simulink model "sedemo_ethernet"  (Simulink 7.5)
settings: Solver=VariableStepDiscrete  StartTime=0.0  StopTime=10.0  MaxStep=inf  RelTol=1e-3
PreLoadFcn:
  | MACInputSize = 25;
  | warning('off','MATLAB:divideByZero');
undefined symbols (not defined in the file or in its folder): des_subsystemblock, des_subsysteminport, des_subsystemoutport, des_subsystemsupportblock
libraries: simeventsrouting1 x30, simeventstranslate1 x26, simeventsattributes2 x16, simeventssink1 x13, simeventsserver1 x13, simeventsgenerators1 x11, simeventssignalmanage1 x9, simeventsgates1 x6, simeventsqueue1 x3, simeventsinfo x1
(part 2 of 5)

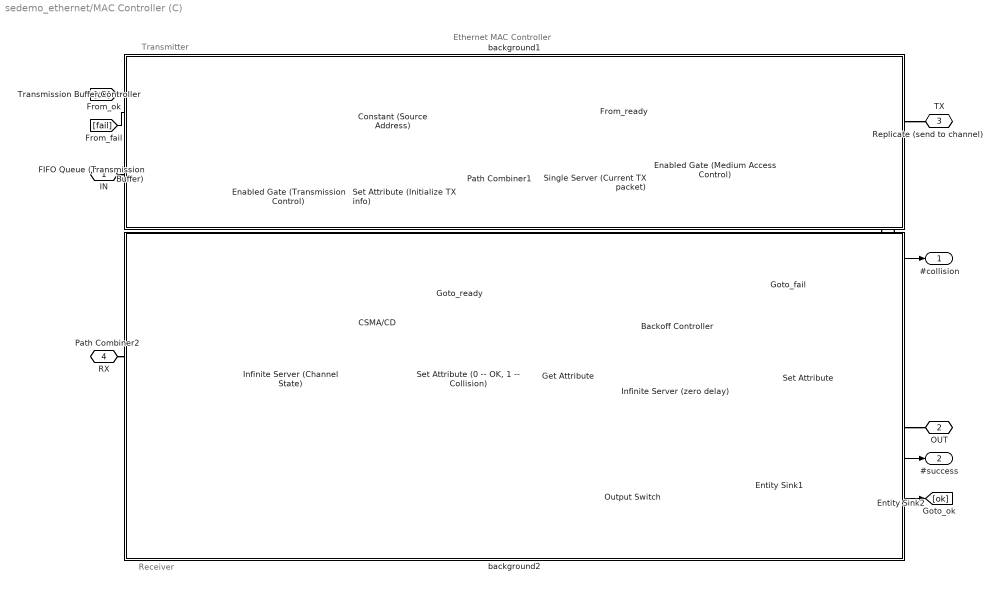
== system sedemo_ethernet/MAC Controller (C) ==
  note: Receiver
  note: Transmitter
  note: Ethernet MAC Controller
  Backoff Controller : Subsystem  LoadFcn=des_subsystemblock(gcb, 'load');  InitFcn=des_subsystemblock(gcb, 'init');  StartFcn=des_subsystemblock(gcb, 'start');  StopFcn=des_subsystemblock(gcb, 'stop');
      settings: CopyFcn=des_subsystemblock(gcb, 'copy');  DeleteFcn=des_subsystemblock(gcb, 'delete');  UndoDeleteFcn=des_subsystemblock(gcb, 'undodelete');  ModelCloseFcn=des_subsystemblock(gcb, 'modelclose');  PreSaveFcn=des_subsystemblock(gcb, 'presave');  NameChangeFcn=des_subsystemblock(gcb, 'namechange');  ParentCloseFcn=des_subsystemblock(gcb, 'parentclose');  ErrorFcn=des_error_redirect
  CSMA/CD : Subsystem
  Constant (Source Address) : Constant  Value=SrcAddress  OutDataType=sfix(16)  OutScaling=2^0
  Enabled Gate (Medium Access Control) : simeventsgates1/Enabled Gate  Priority=1  SystemSampleTime=-1  SpecifyEventPriority=off  PriorityGateEnableOpenClose=200  StatNumberDeparted=Off
  Enabled Gate (Transmission Control) : simeventsgates1/Enabled Gate  Priority=1  SystemSampleTime=-1  SpecifyEventPriority=off  PriorityGateEnableOpenClose=200  StatNumberDeparted=On
  Entity Sink1 : simeventssink1/Entity Sink  Priority=1  SystemSampleTime=-1  AvailableForArrivals=on  StatNumberArrived=On
  Entity Sink2 : simeventssink1/Entity Sink  Priority=1  SystemSampleTime=-1  AvailableForArrivals=on  StatNumberArrived=Off
  FIFO Queue (Transmission Buffer) : simeventsqueue1/FIFO Queue  Priority=1  SystemSampleTime=-1  Capacity=MACInputSize  EnableTOPort=off  StatNumberDeparted=Off  StatNumberInBlock=Off  StatPendingEntity=Off  StatAverageWait=Off  StatAverageQueueLength=Off  StatNumberTimedout=Off
  Get Attribute : simeventsattributes2/Get Attribute  Priority=1  DialogController=des_ddg_create  DialogControllerArgs=DataTag199  SystemSampleTime=-1  AttributeName=SrcAddress|NumCollision|Collision  AttributeMissing=Error|Error|Error  AttributeDefaultValue=0|0|0  AttributeSendTiming=After entity departure|After entity departure|After entity departure  AttributeTreatAsVector=1|1|1  StatNumberDeparted=Off  EvaluatedDefaultAttributeValue={[];[];[]}
  Infinite Server (Channel State) : simeventsserver1/Infinite Server  Priority=1  SystemSampleTime=-1  ServiceTimeFrom=Attribute  ServiceTime=1  AttributeName=ServiceTime  PriorityServiceCompletion=500  EnableTOPort=off  StatNumberDeparted=Off  StatNumberInBlock=On  StatPendingEntity=Off  StatNumberPending=Off  StatAverageWait=Off  StatNumberTimedout=Off
  Infinite Server (zero delay) : simeventsserver1/Infinite Server  Priority=1  SystemSampleTime=-1  ServiceTimeFrom=Dialog  ServiceTime=0  AttributeName=ServiceTime  PriorityServiceCompletion=200  EnableTOPort=off  StatNumberDeparted=Off  StatNumberInBlock=Off  StatPendingEntity=Off  StatNumberPending=Off  StatAverageWait=Off  StatNumberTimedout=Off
  Output Switch : simeventsrouting1/Output Switch  Priority=1  SystemSampleTime=-1  NumberOutputPorts=4  SwitchingCriterion=From attribute  InitialSeed=34567  AttributeName=Route  InitialConditionsOpt=off  InitialConditions=1  EntityBufferOpt=off  SpecifyEventPriority=off  PriorityOutputSwitchSelectPort=4100  TimeoutPortOpt=off  StatNumberDeparted=Off  StatNumberTimedOut=Off  StatPendingEntity=Off  StatLastDeparturePort=Off  EvaluatedNumPorts=4
  Path Combiner1 : simeventsrouting1/Path Combiner  Priority=1  SystemSampleTime=-1  NumberInputPorts=2  InputPortPrecedence=IN1 port  InitialSeed=45675  SpecifyEventPriority=off  PriorityPathCombinerPortPrecedenceSelection=4100  StatNumberDeparted=Off  StatLastArrivalPort=Off  EvaluatedNumPorts=2
  Path Combiner2 : simeventsrouting1/Path Combiner  Priority=1  SystemSampleTime=-1  NumberInputPorts=2  InputPortPrecedence=IN1 port  InitialSeed=45675  SpecifyEventPriority=off  PriorityPathCombinerPortPrecedenceSelection=4100  StatNumberDeparted=Off  StatLastArrivalPort=Off  EvaluatedNumPorts=2
  Replicate (send to channel) : simeventsrouting1/Replicate  Priority=1  SystemSampleTime=-1  NumberOutputPorts=2  ReplicateEntityWhen=All entity output ports are not blocked  OutputPortPrecedence=OUT1 port  InitialSeed=56789  ActionUponBlocking=Discard entity  StatNumberArrived=Off  StatNumberDeparted=Off  EvaluatedNumPorts=2
  Set Attribute : simeventsattributes2/Set Attribute  Priority=1  DialogController=des_ddg_create  DialogControllerArgs=DataTag207  SystemSampleTime=-1  AttributeFrom=Signal port|Signal port|Signal port  AttributeName=Route|NumCollision|BckoffTime  AttributeTreatAsVector=1|1|1  AttributeValue=0|0|0  AttributeCreate=on  StatNumberDeparted=Off  EvaluatedAttributeValue={[];[];[]}
  "Set Attribute (0 -- OK, 1 -- Collision)" : simeventsattributes2/Set Attribute  Priority=1  DialogController=des_ddg_create  DialogControllerArgs=DataTag209  SystemSampleTime=-1  AttributeFrom=Signal port  AttributeName=Collision  AttributeTreatAsVector=1  AttributeValue=0  AttributeCreate=on  StatNumberDeparted=Off  EvaluatedAttributeValue={[]}
  Set Attribute (Initialize TX info) : simeventsattributes2/Set Attribute  Priority=1  DialogController=des_ddg_create  DialogControllerArgs=DataTag211  SystemSampleTime=-1  AttributeFrom=Signal port|Dialog|Dialog  AttributeName=SrcAddress|BckoffTime|NumCollision  AttributeTreatAsVector=1|1|1  AttributeValue=0|0|0  AttributeCreate=on  StatNumberDeparted=Off  EvaluatedAttributeValue={[];0;0}
  Single Server (Current TX packet) : simeventsserver1/Single Server  Priority=1  SystemSampleTime=-1  ServiceTimeFrom=Attribute  ServiceTime=0  AttributeName=BckoffTime  PriorityServiceCompletion=500  PermitPreemption=off  SortingAttributeName=PriorityAttributeName  SortingDirection=Ascending  WriteToAttribute=off  ResidualAttributeName=ResidualServiceTime  CreateAttribute=on  EnableTOPort=off  StatNumberDeparted=Off  StatNumberInBlock=Off  StatNumberPreempted=Off  StatPendingEntity=Off  StatAverageWait=Off  StatUtilization=Off  StatNumberTimedout=Off
  Transmission Buffer Controller : Subsystem
  background1 : Subsystem
      mask Display: disp('')
  background2 : Subsystem
      mask Display: disp('')
  IN : PMIOPort  Port=1  Side=Right
  OUT : PMIOPort  Port=2  Side=Right
  TX : PMIOPort  Port=3  Side=Left
  RX : PMIOPort  Port=4  Side=Left
  #collision : Outport  OutDataType=sfix(16)  OutScaling=2^0
  #success : Outport  Port=2  OutDataType=sfix(16)  OutScaling=2^0
  wires:
  CSMA/CD/1(l_ready) -> [rdy]
  Backoff Controller/2(#failure) -> [fail]
  [fail] -> Transmission Buffer Controller/3(#failure)
  [ok] -> Transmission Buffer Controller/2(#success)
  [rdy] -> Enabled Gate (Medium Access Control)/1
  Backoff Controller/3(route) -> Set Attribute/1
  Backoff Controller/4(#collision1) -> Set Attribute/2
  Backoff Controller/5(bckoffTime) -> Set Attribute/3
  Backoff Controller/1(#sum) -> #collision/1
  Get Attribute/2 -> Backoff Controller/2(#collision)
  Get Attribute/3 -> Backoff Controller/3(collision)
  Get Attribute/1 -> Backoff Controller/1(SrcAddr)
  Constant (Source Address)/1 -> Set Attribute (Initialize TX info)/1
  Transmission Buffer Controller/1(state) -> Enabled Gate (Transmission Control)/1
  CSMA/CD/2(pck_ok) -> "Set Attribute (0 -- OK, 1 -- Collision)"/1
  Entity Sink1/1 -> [ok], #success/1
  Infinite Server (Channel State)/1 -> CSMA/CD/1(l_status)
  Enabled Gate (Transmission Control)/1 -> Transmission Buffer Controller/1(#tx)
  connections:
  Output Switch/RConn4 -- Path Combiner1/LConn1
  Output Switch/RConn1 -- OUT/RConn1
  Set Attribute/RConn1 -- Output Switch/LConn1
  "Set Attribute (0 -- OK, 1 -- Collision)"/RConn1 -- Get Attribute/LConn1
  Infinite Server (zero delay)/RConn1 -- Set Attribute/LConn1
  Get Attribute/RConn1 -- Infinite Server (zero delay)/LConn1
  Output Switch/RConn2 -- Entity Sink1/LConn1
  Output Switch/RConn3 -- Entity Sink2/LConn1
  Enabled Gate (Transmission Control)/RConn1 -- Set Attribute (Initialize TX info)/LConn1
  Set Attribute (Initialize TX info)/RConn1 -- Path Combiner1/LConn2
  Replicate (send to channel)/RConn1 -- TX/RConn1
  FIFO Queue (Transmission Buffer)/RConn1 -- Enabled Gate (Transmission Control)/LConn1
  Replicate (send to channel)/RConn2 -- Path Combiner2/LConn1
  Path Combiner1/RConn1 -- Single Server (Current TX packet)/LConn1
  RX/RConn1 -- Path Combiner2/LConn2
  Enabled Gate (Medium Access Control)/RConn1 -- Replicate (send to channel)/LConn1
  IN/RConn1 -- FIFO Queue (Transmission Buffer)/LConn1
  Infinite Server (Channel State)/RConn1 -- "Set Attribute (0 -- OK, 1 -- Collision)"/LConn1
  Path Combiner2/RConn1 -- Infinite Server (Channel State)/LConn1
  Single Server (Current TX packet)/RConn1 -- Enabled Gate (Medium Access Control)/LConn1

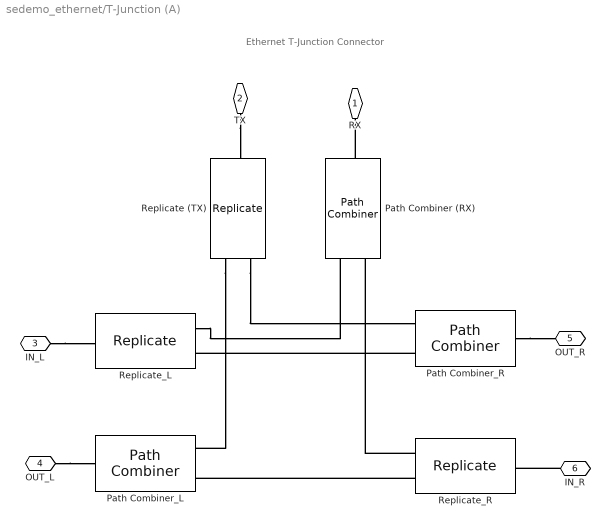
== system sedemo_ethernet/T-Junction (A) ==
  note: Ethernet T-Junction Connector
  Path Combiner (RX) : simeventsrouting1/Path Combiner  Priority=1  SystemSampleTime=-1  NumberInputPorts=2  InputPortPrecedence=IN1 port  InitialSeed=45675  SpecifyEventPriority=off  PriorityPathCombinerPortPrecedenceSelection=4100  StatNumberDeparted=Off  StatLastArrivalPort=Off  EvaluatedNumPorts=2
  Path Combiner_L : simeventsrouting1/Path Combiner  Priority=1  SystemSampleTime=-1  NumberInputPorts=2  InputPortPrecedence=IN1 port  InitialSeed=45675  SpecifyEventPriority=off  PriorityPathCombinerPortPrecedenceSelection=4100  StatNumberDeparted=Off  StatLastArrivalPort=Off  EvaluatedNumPorts=2
  Path Combiner_R : simeventsrouting1/Path Combiner  Priority=1  SystemSampleTime=-1  NumberInputPorts=2  InputPortPrecedence=IN1 port  InitialSeed=45675  SpecifyEventPriority=off  PriorityPathCombinerPortPrecedenceSelection=4100  StatNumberDeparted=Off  StatLastArrivalPort=Off  EvaluatedNumPorts=2
  Replicate (TX) : simeventsrouting1/Replicate  Priority=1  SystemSampleTime=-1  NumberOutputPorts=2  ReplicateEntityWhen=All entity output ports are not blocked  OutputPortPrecedence=OUT1 port  InitialSeed=56789  ActionUponBlocking=Discard entity  StatNumberArrived=Off  StatNumberDeparted=Off  EvaluatedNumPorts=2
  Replicate_L : simeventsrouting1/Replicate  Priority=1  SystemSampleTime=-1  NumberOutputPorts=2  ReplicateEntityWhen=All entity output ports are not blocked  OutputPortPrecedence=OUT1 port  InitialSeed=56789  ActionUponBlocking=Discard entity  StatNumberArrived=Off  StatNumberDeparted=Off  EvaluatedNumPorts=2
  Replicate_R : simeventsrouting1/Replicate  Priority=1  SystemSampleTime=-1  NumberOutputPorts=2  ReplicateEntityWhen=All entity output ports are not blocked  OutputPortPrecedence=OUT1 port  InitialSeed=56789  ActionUponBlocking=Discard entity  StatNumberArrived=Off  StatNumberDeparted=Off  EvaluatedNumPorts=2
  RX : PMIOPort  Port=1  Side=Right
  TX : PMIOPort  Port=2  Side=Left
  IN_L : PMIOPort  Port=3  Side=Left
  OUT_L : PMIOPort  Port=4  Side=Left
  OUT_R : PMIOPort  Port=5  Side=Right
  IN_R : PMIOPort  Port=6  Side=Right
  connections:
  Replicate (TX)/RConn1 -- Path Combiner_L/LConn1
  Replicate (TX)/RConn2 -- Path Combiner_R/LConn1
  TX/RConn1 -- Replicate (TX)/LConn1
  Path Combiner (RX)/RConn1 -- RX/RConn1
  Replicate_R/RConn2 -- Path Combiner_L/LConn2
  OUT_L/RConn1 -- Path Combiner_L/RConn1
  Replicate_R/RConn1 -- Path Combiner (RX)/LConn2
  Replicate_L/RConn1 -- Path Combiner (RX)/LConn1
  IN_R/RConn1 -- Replicate_R/LConn1
  Path Combiner_R/LConn2 -- Replicate_L/RConn2
  IN_L/RConn1 -- Replicate_L/LConn1
  Path Combiner_R/RConn1 -- OUT_R/RConn1

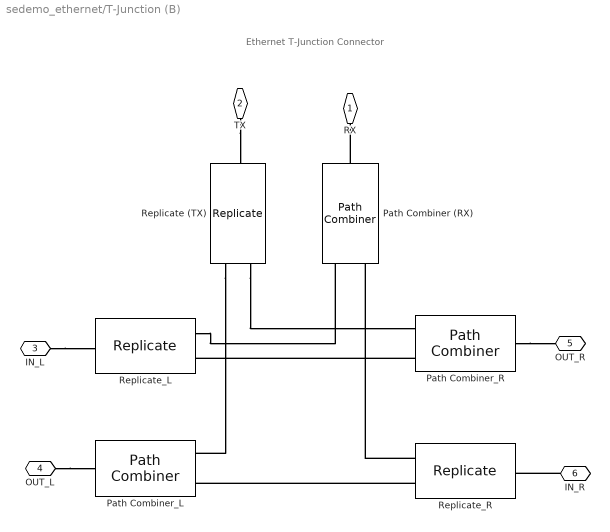
== system sedemo_ethernet/T-Junction (B) ==
  note: Ethernet T-Junction Connector
  Path Combiner (RX) : simeventsrouting1/Path Combiner  Priority=1  SystemSampleTime=-1  NumberInputPorts=2  InputPortPrecedence=IN1 port  InitialSeed=45675  SpecifyEventPriority=off  PriorityPathCombinerPortPrecedenceSelection=4100  StatNumberDeparted=Off  StatLastArrivalPort=Off  EvaluatedNumPorts=2
  Path Combiner_L : simeventsrouting1/Path Combiner  Priority=1  SystemSampleTime=-1  NumberInputPorts=2  InputPortPrecedence=IN1 port  InitialSeed=45675  SpecifyEventPriority=off  PriorityPathCombinerPortPrecedenceSelection=4100  StatNumberDeparted=Off  StatLastArrivalPort=Off  EvaluatedNumPorts=2
  Path Combiner_R : simeventsrouting1/Path Combiner  Priority=1  SystemSampleTime=-1  NumberInputPorts=2  InputPortPrecedence=IN1 port  InitialSeed=45675  SpecifyEventPriority=off  PriorityPathCombinerPortPrecedenceSelection=4100  StatNumberDeparted=Off  StatLastArrivalPort=Off  EvaluatedNumPorts=2
  Replicate (TX) : simeventsrouting1/Replicate  Priority=1  SystemSampleTime=-1  NumberOutputPorts=2  ReplicateEntityWhen=All entity output ports are not blocked  OutputPortPrecedence=OUT1 port  InitialSeed=56789  ActionUponBlocking=Discard entity  StatNumberArrived=Off  StatNumberDeparted=Off  EvaluatedNumPorts=2
  Replicate_L : simeventsrouting1/Replicate  Priority=1  SystemSampleTime=-1  NumberOutputPorts=2  ReplicateEntityWhen=All entity output ports are not blocked  OutputPortPrecedence=OUT1 port  InitialSeed=56789  ActionUponBlocking=Discard entity  StatNumberArrived=Off  StatNumberDeparted=Off  EvaluatedNumPorts=2
  Replicate_R : simeventsrouting1/Replicate  Priority=1  SystemSampleTime=-1  NumberOutputPorts=2  ReplicateEntityWhen=All entity output ports are not blocked  OutputPortPrecedence=OUT1 port  InitialSeed=56789  ActionUponBlocking=Discard entity  StatNumberArrived=Off  StatNumberDeparted=Off  EvaluatedNumPorts=2
  RX : PMIOPort  Port=1  Side=Right
  TX : PMIOPort  Port=2  Side=Left
  IN_L : PMIOPort  Port=3  Side=Left
  OUT_L : PMIOPort  Port=4  Side=Left
  OUT_R : PMIOPort  Port=5  Side=Right
  IN_R : PMIOPort  Port=6  Side=Right
  connections:
  Path Combiner_R/RConn1 -- OUT_R/RConn1
  IN_L/RConn1 -- Replicate_L/LConn1
  Path Combiner_R/LConn2 -- Replicate_L/RConn2
  IN_R/RConn1 -- Replicate_R/LConn1
  Replicate_L/RConn1 -- Path Combiner (RX)/LConn1
  Replicate_R/RConn1 -- Path Combiner (RX)/LConn2
  OUT_L/RConn1 -- Path Combiner_L/RConn1
  Replicate_R/RConn2 -- Path Combiner_L/LConn2
  Path Combiner (RX)/RConn1 -- RX/RConn1
  TX/RConn1 -- Replicate (TX)/LConn1
  Replicate (TX)/RConn2 -- Path Combiner_R/LConn1
  Replicate (TX)/RConn1 -- Path Combiner_L/LConn1

== system sedemo_ethernet/T-Junction (C) ==
  note: Ethernet T-Junction Connector
  Path Combiner (RX) : simeventsrouting1/Path Combiner  Priority=1  SystemSampleTime=-1  NumberInputPorts=2  InputPortPrecedence=IN1 port  InitialSeed=45675  SpecifyEventPriority=off  PriorityPathCombinerPortPrecedenceSelection=4100  StatNumberDeparted=Off  StatLastArrivalPort=Off  EvaluatedNumPorts=2
  Path Combiner_L : simeventsrouting1/Path Combiner  Priority=1  SystemSampleTime=-1  NumberInputPorts=2  InputPortPrecedence=IN1 port  InitialSeed=45675  SpecifyEventPriority=off  PriorityPathCombinerPortPrecedenceSelection=4100  StatNumberDeparted=Off  StatLastArrivalPort=Off  EvaluatedNumPorts=2
  Path Combiner_R : simeventsrouting1/Path Combiner  Priority=1  SystemSampleTime=-1  NumberInputPorts=2  InputPortPrecedence=IN1 port  InitialSeed=45675  SpecifyEventPriority=off  PriorityPathCombinerPortPrecedenceSelection=4100  StatNumberDeparted=Off  StatLastArrivalPort=Off  EvaluatedNumPorts=2
  Replicate (TX) : simeventsrouting1/Replicate  Priority=1  SystemSampleTime=-1  NumberOutputPorts=2  ReplicateEntityWhen=All entity output ports are not blocked  OutputPortPrecedence=OUT1 port  InitialSeed=56789  ActionUponBlocking=Discard entity  StatNumberArrived=Off  StatNumberDeparted=Off  EvaluatedNumPorts=2
  Replicate_L : simeventsrouting1/Replicate  Priority=1  SystemSampleTime=-1  NumberOutputPorts=2  ReplicateEntityWhen=All entity output ports are not blocked  OutputPortPrecedence=OUT1 port  InitialSeed=56789  ActionUponBlocking=Discard entity  StatNumberArrived=Off  StatNumberDeparted=Off  EvaluatedNumPorts=2
  Replicate_R : simeventsrouting1/Replicate  Priority=1  SystemSampleTime=-1  NumberOutputPorts=2  ReplicateEntityWhen=All entity output ports are not blocked  OutputPortPrecedence=OUT1 port  InitialSeed=56789  ActionUponBlocking=Discard entity  StatNumberArrived=Off  StatNumberDeparted=Off  EvaluatedNumPorts=2
  RX : PMIOPort  Port=1  Side=Right
  TX : PMIOPort  Port=2  Side=Left
  IN_L : PMIOPort  Port=3  Side=Left
  OUT_L : PMIOPort  Port=4  Side=Left
  OUT_R : PMIOPort  Port=5  Side=Right
  IN_R : PMIOPort  Port=6  Side=Right
  connections:
  Path Combiner_R/RConn1 -- OUT_R/RConn1
  IN_L/RConn1 -- Replicate_L/LConn1
  Path Combiner_R/LConn2 -- Replicate_L/RConn2
  IN_R/RConn1 -- Replicate_R/LConn1
  Replicate_L/RConn1 -- Path Combiner (RX)/LConn1
  Replicate_R/RConn1 -- Path Combiner (RX)/LConn2
  OUT_L/RConn1 -- Path Combiner_L/RConn1
  Replicate_R/RConn2 -- Path Combiner_L/LConn2
  Path Combiner (RX)/RConn1 -- RX/RConn1
  TX/RConn1 -- Replicate (TX)/LConn1
  Replicate (TX)/RConn2 -- Path Combiner_R/LConn1
  Replicate (TX)/RConn1 -- Path Combiner_L/LConn1

== system sedemo_ethernet/Terminator (L) ==
  note: Ethernet Terminator
  Entity Sink : simeventssink1/Entity Sink  Priority=1  SystemSampleTime=-1  AvailableForArrivals=on  StatNumberArrived=Off
  Event-Based Entity Generator : simeventsgenerators1/Entity Generators/Event-Based Entity Generator  Priority=1  DialogController=des_ddg_create  DialogControllerArgs=DataTag244  SystemSampleTime=-1  GenerateEntitiesUpon=Change in signal from port vc  SignalEdgeType=Rising  SpecifyEventPriority=off  PriorityEntityGeneration=300  GenerateEntityAtSimulationStart=on  AllowBlocking=on  ResponseDuringBlockage=Discard generated entities  EntityType=Standard  StatNumberDeparted=Off  StatPendingEntity=Off  StatAverageIntergenerationTime=Off
  Ground : Ground
  OUT : PMIOPort  Port=1  Side=Left
  IN : PMIOPort  Port=2  Side=Left
  wires:
  Ground/1 -> Event-Based Entity Generator/1
  connections:
  Event-Based Entity Generator/RConn1 -- OUT/RConn1
  IN/RConn1 -- Entity Sink/LConn1

== system sedemo_ethernet/Terminator (R) ==
  Entity Sink : simeventssink1/Entity Sink  Priority=1  SystemSampleTime=-1  AvailableForArrivals=on  StatNumberArrived=Off
  Event-Based Entity Generator : simeventsgenerators1/Entity Generators/Event-Based Entity Generator  Priority=1  DialogController=des_ddg_create  DialogControllerArgs=DataTag247  SystemSampleTime=-1  GenerateEntitiesUpon=Change in signal from port vc  SignalEdgeType=Rising  SpecifyEventPriority=off  PriorityEntityGeneration=300  GenerateEntityAtSimulationStart=on  AllowBlocking=on  ResponseDuringBlockage=Discard generated entities  EntityType=Standard  StatNumberDeparted=Off  StatPendingEntity=Off  StatAverageIntergenerationTime=Off
  Ground : Ground
  IN : PMIOPort  Port=1  Side=Left
  OUT : PMIOPort  Port=2  Side=Left
  wires:
  Ground/1 -> Event-Based Entity Generator/1
  connections:
  Event-Based Entity Generator/RConn1 -- OUT/RConn1
  IN/RConn1 -- Entity Sink/LConn1

== system sedemo_ethernet/Application (A)/Compute comm delay ==
  note: PLEASE DO NOT MODIFY ANYTHING IN THIS SUBSYSTEM.
      | This Subsystem is automatically generated and
      | managed by the Discrete Event Subsystem.
  size : Inport  DataType=double  OutDataType=sfix(16)  OutScaling=2^0  OutDataTypeStr=double
  AAA___ : Subsystem  LoadFcn=des_subsystemsupportblock(gcb, 'load');  InitFcn=des_subsystemsupportblock(gcb, 'init');  StartFcn=des_subsystemsupportblock(gcb, 'start');  StopFcn=des_subsystemsupportblock(gcb, 'stop');
      settings: CopyFcn=des_subsystemsupportblock(gcb, 'copy');  DeleteFcn=des_subsystemsupportblock(gcb, 'delete');  UndoDeleteFcn=des_subsystemsupportblock(gcb, 'undodelete');  ModelCloseFcn=des_subsystemsupportblock(gcb, 'modelclose');  PreSaveFcn=des_subsystemsupportblock(gcb, 'presave');  NameChangeFcn=des_subsystemsupportblock(gcb, 'namechange');  OpenFcn=des_subsystemsupportblock(gcb, 'open');  ParentCloseFcn=des_subsystemsupportblock(gcb, 'parentclose');
  Mux : Mux  Inputs=1
  __fcn_ss__ : Subsystem  TreatAsAtomicUnit=on
      settings: PropExecContextOutsideSubsystem=on
  c_size : Constant  OutDataType=sfix(16)  OutScaling=2^0
  f_size : simeventstranslate1/Signal-Based Event to Function-Call Event  Priority=1  SystemSampleTime=-1  GenerateFunctionCallUpon=Sample time hit from port ts  SignalEdgeOption=Rising  EnableE1Port=on  EnableF2Port=off  EnableE2Port=off  SpecifyEventPriority=off  PriorityFunctionCall=20  FunctionCallDelayFrom=Dialog  DelayFunctionCall=0  StatNumberF1Calls=Off  StatNumberF2Calls=Off  MaskBlockType=DESS_EVENT_PORT
  delay : Outport  OutDataType=sfix(16)  OutScaling=2^0
  wires:
  size/1 -> __fcn_ss__/1(size), f_size/1
  Mux/1 -> __fcn_ss__/Trigger
  c_size/1 -> f_size/2
  f_size/1 -> Mux/1
  __fcn_ss__/1(delay) -> delay/1

== system sedemo_ethernet/Application (B)/Compute comm delay ==
  note: PLEASE DO NOT MODIFY ANYTHING IN THIS SUBSYSTEM.
      | This Subsystem is automatically generated and
      | managed by the Discrete Event Subsystem.
  size : Inport  DataType=double  OutDataType=sfix(16)  OutScaling=2^0  OutDataTypeStr=double
  AAA___ : Subsystem  LoadFcn=des_subsystemsupportblock(gcb, 'load');  InitFcn=des_subsystemsupportblock(gcb, 'init');  StartFcn=des_subsystemsupportblock(gcb, 'start');  StopFcn=des_subsystemsupportblock(gcb, 'stop');
      settings: CopyFcn=des_subsystemsupportblock(gcb, 'copy');  DeleteFcn=des_subsystemsupportblock(gcb, 'delete');  UndoDeleteFcn=des_subsystemsupportblock(gcb, 'undodelete');  ModelCloseFcn=des_subsystemsupportblock(gcb, 'modelclose');  PreSaveFcn=des_subsystemsupportblock(gcb, 'presave');  NameChangeFcn=des_subsystemsupportblock(gcb, 'namechange');  OpenFcn=des_subsystemsupportblock(gcb, 'open');  ParentCloseFcn=des_subsystemsupportblock(gcb, 'parentclose');
  Mux : Mux  Inputs=1
  __fcn_ss__ : Subsystem  TreatAsAtomicUnit=on
      settings: PropExecContextOutsideSubsystem=on
  c_size : Constant  OutDataType=sfix(16)  OutScaling=2^0
  f_size : simeventstranslate1/Signal-Based Event to Function-Call Event  Priority=1  SystemSampleTime=-1  GenerateFunctionCallUpon=Sample time hit from port ts  SignalEdgeOption=Rising  EnableE1Port=on  EnableF2Port=off  EnableE2Port=off  SpecifyEventPriority=off  PriorityFunctionCall=20  FunctionCallDelayFrom=Dialog  DelayFunctionCall=0  StatNumberF1Calls=Off  StatNumberF2Calls=Off  MaskBlockType=DESS_EVENT_PORT
  delay : Outport  OutDataType=sfix(16)  OutScaling=2^0
  wires:
  size/1 -> __fcn_ss__/1(size), f_size/1
  Mux/1 -> __fcn_ss__/Trigger
  c_size/1 -> f_size/2
  f_size/1 -> Mux/1
  __fcn_ss__/1(delay) -> delay/1

== system sedemo_ethernet/Application (C)/Compute comm delay ==
  note: PLEASE DO NOT MODIFY ANYTHING IN THIS SUBSYSTEM.
      | This Subsystem is automatically generated and
      | managed by the Discrete Event Subsystem.
  size : Inport  DataType=double  OutDataType=sfix(16)  OutScaling=2^0  OutDataTypeStr=double
  AAA___ : Subsystem  LoadFcn=des_subsystemsupportblock(gcb, 'load');  InitFcn=des_subsystemsupportblock(gcb, 'init');  StartFcn=des_subsystemsupportblock(gcb, 'start');  StopFcn=des_subsystemsupportblock(gcb, 'stop');
      settings: CopyFcn=des_subsystemsupportblock(gcb, 'copy');  DeleteFcn=des_subsystemsupportblock(gcb, 'delete');  UndoDeleteFcn=des_subsystemsupportblock(gcb, 'undodelete');  ModelCloseFcn=des_subsystemsupportblock(gcb, 'modelclose');  PreSaveFcn=des_subsystemsupportblock(gcb, 'presave');  NameChangeFcn=des_subsystemsupportblock(gcb, 'namechange');  OpenFcn=des_subsystemsupportblock(gcb, 'open');  ParentCloseFcn=des_subsystemsupportblock(gcb, 'parentclose');
  Mux : Mux  Inputs=1
  __fcn_ss__ : Subsystem  TreatAsAtomicUnit=on
      settings: PropExecContextOutsideSubsystem=on
  c_size : Constant  OutDataType=sfix(16)  OutScaling=2^0
  f_size : simeventstranslate1/Signal-Based Event to Function-Call Event  Priority=1  SystemSampleTime=-1  GenerateFunctionCallUpon=Sample time hit from port ts  SignalEdgeOption=Rising  EnableE1Port=on  EnableF2Port=off  EnableE2Port=off  SpecifyEventPriority=off  PriorityFunctionCall=20  FunctionCallDelayFrom=Dialog  DelayFunctionCall=0  StatNumberF1Calls=Off  StatNumberF2Calls=Off  MaskBlockType=DESS_EVENT_PORT
  delay : Outport  OutDataType=sfix(16)  OutScaling=2^0
  wires:
  size/1 -> __fcn_ss__/1(size), f_size/1
  Mux/1 -> __fcn_ss__/Trigger
  c_size/1 -> f_size/2
  f_size/1 -> Mux/1
  __fcn_ss__/1(delay) -> delay/1

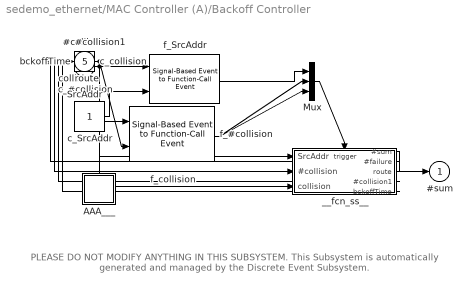
== system sedemo_ethernet/MAC Controller (A)/Backoff Controller ==
  note: PLEASE DO NOT MODIFY ANYTHING IN THIS SUBSYSTEM.
      | This Subsystem is automatically generated and
      | managed by the Discrete Event Subsystem.
  SrcAddr : Inport  DataType=double  OutDataType=sfix(16)  OutScaling=2^0  OutDataTypeStr=double
  #collision : Inport  Port=2  DataType=double  OutDataType=sfix(16)  OutScaling=2^0  OutDataTypeStr=double
  collision : Inport  Port=3  DataType=double  OutDataType=sfix(16)  OutScaling=2^0  OutDataTypeStr=double
  AAA___ : Subsystem  LoadFcn=des_subsystemsupportblock(gcb, 'load');  InitFcn=des_subsystemsupportblock(gcb, 'init');  StartFcn=des_subsystemsupportblock(gcb, 'start');  StopFcn=des_subsystemsupportblock(gcb, 'stop');
      settings: CopyFcn=des_subsystemsupportblock(gcb, 'copy');  DeleteFcn=des_subsystemsupportblock(gcb, 'delete');  UndoDeleteFcn=des_subsystemsupportblock(gcb, 'undodelete');  ModelCloseFcn=des_subsystemsupportblock(gcb, 'modelclose');  PreSaveFcn=des_subsystemsupportblock(gcb, 'presave');  NameChangeFcn=des_subsystemsupportblock(gcb, 'namechange');  OpenFcn=des_subsystemsupportblock(gcb, 'open');  ParentCloseFcn=des_subsystemsupportblock(gcb, 'parentclose');
  Mux : Mux  Inputs=3
  __fcn_ss__ : Subsystem  TreatAsAtomicUnit=on
      settings: PropExecContextOutsideSubsystem=on
  c_#collision : Constant  Value=0  OutDataType=sfix(16)  OutScaling=2^0
  c_SrcAddr : Constant  OutDataType=sfix(16)  OutScaling=2^0
  c_collision : Constant  Value=0  OutDataType=sfix(16)  OutScaling=2^0
  f_#collision : simeventstranslate1/Signal-Based Event to Function-Call Event  Priority=1  SystemSampleTime=-1  GenerateFunctionCallUpon=Sample time hit from port ts  SignalEdgeOption=Rising  EnableE1Port=on  EnableF2Port=off  EnableE2Port=off  SpecifyEventPriority=off  PriorityFunctionCall=20  FunctionCallDelayFrom=Dialog  DelayFunctionCall=0  StatNumberF1Calls=Off  StatNumberF2Calls=Off  MaskBlockType=DESS_DATA_PORT
  f_SrcAddr : simeventstranslate1/Signal-Based Event to Function-Call Event  Priority=1  SystemSampleTime=-1  GenerateFunctionCallUpon=Sample time hit from port ts  SignalEdgeOption=Rising  EnableE1Port=on  EnableF2Port=off  EnableE2Port=off  SpecifyEventPriority=on  PriorityFunctionCall=20  FunctionCallDelayFrom=Dialog  DelayFunctionCall=0  StatNumberF1Calls=Off  StatNumberF2Calls=Off  MaskBlockType=DESS_EVENT_PORT
  f_collision : simeventstranslate1/Signal-Based Event to Function-Call Event  Priority=1  SystemSampleTime=-1  GenerateFunctionCallUpon=Sample time hit from port ts  SignalEdgeOption=Rising  EnableE1Port=on  EnableF2Port=off  EnableE2Port=off  SpecifyEventPriority=off  PriorityFunctionCall=200  FunctionCallDelayFrom=Dialog  DelayFunctionCall=0  StatNumberF1Calls=Off  StatNumberF2Calls=Off  MaskBlockType=DESS_DATA_PORT
  #sum : Outport  OutDataType=sfix(16)  OutScaling=2^0
  #failure : Outport  Port=2  OutDataType=sfix(16)  OutScaling=2^0
  route : Outport  Port=3  OutDataType=sfix(16)  OutScaling=2^0
  #collision1 : Outport  Port=4  OutDataType=sfix(16)  OutScaling=2^0
  bckoffTime : Outport  Port=5  OutDataType=sfix(16)  OutScaling=2^0
  wires:
  SrcAddr/1 -> __fcn_ss__/1(SrcAddr), f_SrcAddr/1
  __fcn_ss__/5(bckoffTime) -> bckoffTime/1
  c_collision/1 -> f_collision/2
  f_collision/1 -> Mux/3
  collision/1 -> __fcn_ss__/3(collision), f_collision/1
  __fcn_ss__/4(#collision1) -> #collision1/1
  __fcn_ss__/3(route) -> route/1
  __fcn_ss__/2(#failure) -> #failure/1
  #collision/1 -> __fcn_ss__/2(#collision), f_#collision/1
  c_#collision/1 -> f_#collision/2
  f_#collision/1 -> Mux/2
  Mux/1 -> __fcn_ss__/Trigger
  c_SrcAddr/1 -> f_SrcAddr/2
  f_SrcAddr/1 -> Mux/1
  __fcn_ss__/1(#sum) -> #sum/1

== system sedemo_ethernet/MAC Controller (A)/CSMA/CD ==
  note: Carrier Sense Multiple Access with Collision Detection
  note: This subsystem aims to determine whether a packet is the only packet on the communication channel for the entire duration of transmission.
      |
      | The l_status input signal is the number of packets in a server in the parent system (Ethernet MAC Controller). The Signal Latch block responds
      | to these events:
      |
      |     -- If l_status increases from 0 to 1, then
      |        -- rtr has a rising edge.
      |        -- The Signal Latch block processes a read event.
      |        -- The Signal Latch block's st output signal becomes 0.
      |
      |     -- If l_status increases from 1 to 2, then
      |         -- wtr has a rising edge.
      |         -- The Signal Latch block processes a write event.
      |         -- The Signal Latch block's st output signal becomes 1.
      |
      | By the time the packet departs from the server in the parent system, the Signal Latch block's st signal is 0 if and only if that packet has been the
      | only packet in the server block for the entire duration of service. This outcome respresents a success for that packet. Other outcomes represent
      | collisions between that packet and one or more other packets.
  l_status : Inport  OutDataType=sfix(16)  OutScaling=2^0
  Discrete Event Subsystem (Carrier Sensing) : Subsystem  LoadFcn=des_subsystemblock(gcb, 'load');  InitFcn=des_subsystemblock(gcb, 'init');  StartFcn=des_subsystemblock(gcb, 'start');  StopFcn=des_subsystemblock(gcb, 'stop');
      settings: CopyFcn=des_subsystemblock(gcb, 'copy');  DeleteFcn=des_subsystemblock(gcb, 'delete');  UndoDeleteFcn=des_subsystemblock(gcb, 'undodelete');  ModelCloseFcn=des_subsystemblock(gcb, 'modelclose');  PreSaveFcn=des_subsystemblock(gcb, 'presave');  NameChangeFcn=des_subsystemblock(gcb, 'namechange');  ParentCloseFcn=des_subsystemblock(gcb, 'parentclose');  ErrorFcn=des_error_redirect
  Ground : Ground
  Signal Latch (Collision Detection) : simeventssignalmanage1/Signal Latch  Priority=1  SystemSampleTime=-1  InitialMemoryValue=0  WriteMemoryUpon=Trigger from port wtr  MemoryWriteEdgeOption=Rising  SpecifyWriteEventPriority=on  PriorityMemoryWrite=7100  ReadMemoryUpon=Trigger from port rtr  MemoryReadEdgeOption=Rising  SpecifyReadEventPriority=on  PriorityMemoryRead=7000  ReportMemoryState=on  ReportMemoryUponWrite=off  ReportMemoryUponRead=off
  l_ready : Outport  OutDataType=sfix(16)  OutScaling=2^0
  pck_ok : Outport  Port=2  OutDataType=sfix(16)  OutScaling=2^0
  wires:
  Discrete Event Subsystem (Carrier Sensing)/1(l_ready) -> l_ready/1
  l_status/1 -> Discrete Event Subsystem (Carrier Sensing)/1(l_status), Signal Latch (Collision Detection)/2
  Ground/1 -> Signal Latch (Collision Detection)/3
  Discrete Event Subsystem (Carrier Sensing)/2(collision) -> Signal Latch (Collision Detection)/1
  Signal Latch (Collision Detection)/1 -> pck_ok/1

== system sedemo_ethernet/MAC Controller (A)/Transmission Buffer Controller ==
  #tx : Inport  OutDataType=sfix(16)  OutScaling=2^0
  #success : Inport  Port=2  OutDataType=sfix(16)  OutScaling=2^0
  #failure : Inport  Port=3  OutDataType=sfix(16)  OutScaling=2^0
  Initial Value : simeventssignalmanage1/Initial Value  InitialValue=1
  Transmission Buffer Controller : Subsystem  LoadFcn=des_subsystemblock(gcb, 'load');  InitFcn=des_subsystemblock(gcb, 'init');  StartFcn=des_subsystemblock(gcb, 'start');  StopFcn=des_subsystemblock(gcb, 'stop');
      settings: CopyFcn=des_subsystemblock(gcb, 'copy');  DeleteFcn=des_subsystemblock(gcb, 'delete');  UndoDeleteFcn=des_subsystemblock(gcb, 'undodelete');  ModelCloseFcn=des_subsystemblock(gcb, 'modelclose');  PreSaveFcn=des_subsystemblock(gcb, 'presave');  NameChangeFcn=des_subsystemblock(gcb, 'namechange');  ParentCloseFcn=des_subsystemblock(gcb, 'parentclose');  ErrorFcn=des_error_redirect
  state : Outport  OutDataType=sfix(16)  OutScaling=2^0
  wires:
  Initial Value/1 -> state/1
  Transmission Buffer Controller/1(state) -> Initial Value/1
  #failure/1 -> Transmission Buffer Controller/3(#failure)
  #success/1 -> Transmission Buffer Controller/2(#success)
  #tx/1 -> Transmission Buffer Controller/1(#tx)

== system sedemo_ethernet/MAC Controller (A)/background1 ==

== system sedemo_ethernet/MAC Controller (A)/background2 ==

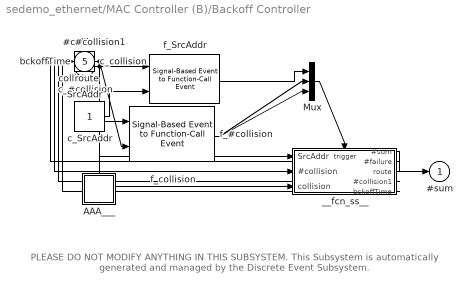
== system sedemo_ethernet/MAC Controller (B)/Backoff Controller ==
  note: PLEASE DO NOT MODIFY ANYTHING IN THIS SUBSYSTEM.
      | This Subsystem is automatically generated and
      | managed by the Discrete Event Subsystem.
  SrcAddr : Inport  DataType=double  OutDataType=sfix(16)  OutScaling=2^0  OutDataTypeStr=double
  #collision : Inport  Port=2  DataType=double  OutDataType=sfix(16)  OutScaling=2^0  OutDataTypeStr=double
  collision : Inport  Port=3  DataType=double  OutDataType=sfix(16)  OutScaling=2^0  OutDataTypeStr=double
  AAA___ : Subsystem  LoadFcn=des_subsystemsupportblock(gcb, 'load');  InitFcn=des_subsystemsupportblock(gcb, 'init');  StartFcn=des_subsystemsupportblock(gcb, 'start');  StopFcn=des_subsystemsupportblock(gcb, 'stop');
      settings: CopyFcn=des_subsystemsupportblock(gcb, 'copy');  DeleteFcn=des_subsystemsupportblock(gcb, 'delete');  UndoDeleteFcn=des_subsystemsupportblock(gcb, 'undodelete');  ModelCloseFcn=des_subsystemsupportblock(gcb, 'modelclose');  PreSaveFcn=des_subsystemsupportblock(gcb, 'presave');  NameChangeFcn=des_subsystemsupportblock(gcb, 'namechange');  OpenFcn=des_subsystemsupportblock(gcb, 'open');  ParentCloseFcn=des_subsystemsupportblock(gcb, 'parentclose');
  Mux : Mux  Inputs=3
  __fcn_ss__ : Subsystem  TreatAsAtomicUnit=on
      settings: PropExecContextOutsideSubsystem=on
  c_#collision : Constant  Value=0  OutDataType=sfix(16)  OutScaling=2^0
  c_SrcAddr : Constant  OutDataType=sfix(16)  OutScaling=2^0
  c_collision : Constant  Value=0  OutDataType=sfix(16)  OutScaling=2^0
  f_#collision : simeventstranslate1/Signal-Based Event to Function-Call Event  Priority=1  SystemSampleTime=-1  GenerateFunctionCallUpon=Sample time hit from port ts  SignalEdgeOption=Rising  EnableE1Port=on  EnableF2Port=off  EnableE2Port=off  SpecifyEventPriority=off  PriorityFunctionCall=20  FunctionCallDelayFrom=Dialog  DelayFunctionCall=0  StatNumberF1Calls=Off  StatNumberF2Calls=Off  MaskBlockType=DESS_DATA_PORT
  f_SrcAddr : simeventstranslate1/Signal-Based Event to Function-Call Event  Priority=1  SystemSampleTime=-1  GenerateFunctionCallUpon=Sample time hit from port ts  SignalEdgeOption=Rising  EnableE1Port=on  EnableF2Port=off  EnableE2Port=off  SpecifyEventPriority=on  PriorityFunctionCall=20  FunctionCallDelayFrom=Dialog  DelayFunctionCall=0  StatNumberF1Calls=Off  StatNumberF2Calls=Off  MaskBlockType=DESS_EVENT_PORT
  f_collision : simeventstranslate1/Signal-Based Event to Function-Call Event  Priority=1  SystemSampleTime=-1  GenerateFunctionCallUpon=Sample time hit from port ts  SignalEdgeOption=Rising  EnableE1Port=on  EnableF2Port=off  EnableE2Port=off  SpecifyEventPriority=off  PriorityFunctionCall=200  FunctionCallDelayFrom=Dialog  DelayFunctionCall=0  StatNumberF1Calls=Off  StatNumberF2Calls=Off  MaskBlockType=DESS_DATA_PORT
  #sum : Outport  OutDataType=sfix(16)  OutScaling=2^0
  #failure : Outport  Port=2  OutDataType=sfix(16)  OutScaling=2^0
  route : Outport  Port=3  OutDataType=sfix(16)  OutScaling=2^0
  #collision1 : Outport  Port=4  OutDataType=sfix(16)  OutScaling=2^0
  bckoffTime : Outport  Port=5  OutDataType=sfix(16)  OutScaling=2^0
  wires:
  SrcAddr/1 -> __fcn_ss__/1(SrcAddr), f_SrcAddr/1
  __fcn_ss__/5(bckoffTime) -> bckoffTime/1
  c_collision/1 -> f_collision/2
  f_collision/1 -> Mux/3
  collision/1 -> __fcn_ss__/3(collision), f_collision/1
  __fcn_ss__/4(#collision1) -> #collision1/1
  __fcn_ss__/3(route) -> route/1
  __fcn_ss__/2(#failure) -> #failure/1
  #collision/1 -> __fcn_ss__/2(#collision), f_#collision/1
  c_#collision/1 -> f_#collision/2
  f_#collision/1 -> Mux/2
  Mux/1 -> __fcn_ss__/Trigger
  c_SrcAddr/1 -> f_SrcAddr/2
  f_SrcAddr/1 -> Mux/1
  __fcn_ss__/1(#sum) -> #sum/1

== system sedemo_ethernet/MAC Controller (B)/CSMA/CD ==
  note: This subsystem aims to determine whether a packet is the only packet on the communication channel for the entire duration of transmission.
      |
      | The l_status input signal is the number of packets in a server in the parent system (Ethernet MAC Controller). The Signal Latch block responds
      | to these events:
      |
      |     -- If l_status increases from 0 to 1, then
      |        -- rtr has a rising edge.
      |        -- The Signal Latch block processes a read event.
      |        -- The Signal Latch block's st output signal becomes 0.
      |
      |     -- If l_status increases from 1 to 2, then
      |         -- wtr has a rising edge.
      |         -- The Signal Latch block processes a write event.
      |         -- The Signal Latch block's st output signal becomes 1.
      |
      | By the time the packet departs from the server in the parent system, the Signal Latch block's st signal is 0 if and only if that packet has been the
      | only packet in the server block for the entire duration of service. This outcome respresents a success for that packet. Other outcomes represent
      | collisions between that packet and one or more other packets.
  note: Carrier Sense Multiple Access with Collision Detection
  l_status : Inport  OutDataType=sfix(16)  OutScaling=2^0
  Discrete Event Subsystem (Carrier Sensing) : Subsystem  LoadFcn=des_subsystemblock(gcb, 'load');  InitFcn=des_subsystemblock(gcb, 'init');  StartFcn=des_subsystemblock(gcb, 'start');  StopFcn=des_subsystemblock(gcb, 'stop');
      settings: CopyFcn=des_subsystemblock(gcb, 'copy');  DeleteFcn=des_subsystemblock(gcb, 'delete');  UndoDeleteFcn=des_subsystemblock(gcb, 'undodelete');  ModelCloseFcn=des_subsystemblock(gcb, 'modelclose');  PreSaveFcn=des_subsystemblock(gcb, 'presave');  NameChangeFcn=des_subsystemblock(gcb, 'namechange');  ParentCloseFcn=des_subsystemblock(gcb, 'parentclose');  ErrorFcn=des_error_redirect
  Ground : Ground
  Signal Latch (Collision Detection) : simeventssignalmanage1/Signal Latch  Priority=1  SystemSampleTime=-1  InitialMemoryValue=0  WriteMemoryUpon=Trigger from port wtr  MemoryWriteEdgeOption=Rising  SpecifyWriteEventPriority=on  PriorityMemoryWrite=7100  ReadMemoryUpon=Trigger from port rtr  MemoryReadEdgeOption=Rising  SpecifyReadEventPriority=on  PriorityMemoryRead=7000  ReportMemoryState=on  ReportMemoryUponWrite=off  ReportMemoryUponRead=off
  l_ready : Outport  OutDataType=sfix(16)  OutScaling=2^0
  pck_ok : Outport  Port=2  OutDataType=sfix(16)  OutScaling=2^0
  wires:
  Discrete Event Subsystem (Carrier Sensing)/1(l_ready) -> l_ready/1
  l_status/1 -> Discrete Event Subsystem (Carrier Sensing)/1(l_status), Signal Latch (Collision Detection)/2
  Ground/1 -> Signal Latch (Collision Detection)/3
  Discrete Event Subsystem (Carrier Sensing)/2(collision) -> Signal Latch (Collision Detection)/1
  Signal Latch (Collision Detection)/1 -> pck_ok/1

== system sedemo_ethernet/MAC Controller (B)/Compute  channel utilization ==
  note: PLEASE DO NOT MODIFY ANYTHING IN THIS SUBSYSTEM.
      | This Subsystem is automatically generated and
      | managed by the Discrete Event Subsystem.
  #n : Inport  DataType=double  OutDataType=sfix(16)  OutScaling=2^0  OutDataTypeStr=double
  AAA___ : Subsystem  LoadFcn=des_subsystemsupportblock(gcb, 'load');  InitFcn=des_subsystemsupportblock(gcb, 'init');  StartFcn=des_subsystemsupportblock(gcb, 'start');  StopFcn=des_subsystemsupportblock(gcb, 'stop');
      settings: CopyFcn=des_subsystemsupportblock(gcb, 'copy');  DeleteFcn=des_subsystemsupportblock(gcb, 'delete');  UndoDeleteFcn=des_subsystemsupportblock(gcb, 'undodelete');  ModelCloseFcn=des_subsystemsupportblock(gcb, 'modelclose');  PreSaveFcn=des_subsystemsupportblock(gcb, 'presave');  NameChangeFcn=des_subsystemsupportblock(gcb, 'namechange');  OpenFcn=des_subsystemsupportblock(gcb, 'open');  ParentCloseFcn=des_subsystemsupportblock(gcb, 'parentclose');
  Mux : Mux  Inputs=2
  __fcn_ss__ : Subsystem  TreatAsAtomicUnit=on
      settings: PropExecContextOutsideSubsystem=on
  c_#n : Constant  OutDataType=sfix(16)  OutScaling=2^0
  f_#n : simeventstranslate1/Signal-Based Event to Function-Call Event  Priority=1  SystemSampleTime=-1  GenerateFunctionCallUpon=Sample time hit from port ts  SignalEdgeOption=Rising  EnableE1Port=on  EnableF2Port=off  EnableE2Port=off  SpecifyEventPriority=off  PriorityFunctionCall=20  FunctionCallDelayFrom=Dialog  DelayFunctionCall=0  StatNumberF1Calls=Off  StatNumberF2Calls=Off  MaskBlockType=DESS_EVENT_PORT
  ground : Ground
  util : Outport  OutDataType=sfix(16)  OutScaling=2^0
  wires:
  #n/1 -> __fcn_ss__/1(#n), f_#n/1
  ground/1 -> Mux/2
  Mux/1 -> __fcn_ss__/Trigger
  c_#n/1 -> f_#n/2
  f_#n/1 -> Mux/1
  __fcn_ss__/1(util) -> util/1

== system sedemo_ethernet/MAC Controller (B)/Compute Tx throughput ==
  note: PLEASE DO NOT MODIFY ANYTHING IN THIS SUBSYSTEM.
      | This Subsystem is automatically generated and
      | managed by the Discrete Event Subsystem.
  PckSize : Inport  DataType=double  OutDataType=sfix(16)  OutScaling=2^0  OutDataTypeStr=double
  AAA___ : Subsystem  LoadFcn=des_subsystemsupportblock(gcb, 'load');  InitFcn=des_subsystemsupportblock(gcb, 'init');  StartFcn=des_subsystemsupportblock(gcb, 'start');  StopFcn=des_subsystemsupportblock(gcb, 'stop');
      settings: CopyFcn=des_subsystemsupportblock(gcb, 'copy');  DeleteFcn=des_subsystemsupportblock(gcb, 'delete');  UndoDeleteFcn=des_subsystemsupportblock(gcb, 'undodelete');  ModelCloseFcn=des_subsystemsupportblock(gcb, 'modelclose');  PreSaveFcn=des_subsystemsupportblock(gcb, 'presave');  NameChangeFcn=des_subsystemsupportblock(gcb, 'namechange');  OpenFcn=des_subsystemsupportblock(gcb, 'open');  ParentCloseFcn=des_subsystemsupportblock(gcb, 'parentclose');
  Mux : Mux  Inputs=2
  __fcn_ss__ : Subsystem  TreatAsAtomicUnit=on
      settings: PropExecContextOutsideSubsystem=on
  c_PckSize : Constant  OutDataType=sfix(16)  OutScaling=2^0
  f_PckSize : simeventstranslate1/Signal-Based Event to Function-Call Event  Priority=1  SystemSampleTime=-1  GenerateFunctionCallUpon=Sample time hit from port ts  SignalEdgeOption=Rising  EnableE1Port=on  EnableF2Port=off  EnableE2Port=off  SpecifyEventPriority=off  PriorityFunctionCall=20  FunctionCallDelayFrom=Dialog  DelayFunctionCall=0  StatNumberF1Calls=Off  StatNumberF2Calls=Off  MaskBlockType=DESS_EVENT_PORT
  ground : Ground
  rate : Outport  OutDataType=sfix(16)  OutScaling=2^0
  wires:
  PckSize/1 -> __fcn_ss__/1(PckSize), f_PckSize/1
  __fcn_ss__/1(rate) -> rate/1
  f_PckSize/1 -> Mux/1
  c_PckSize/1 -> f_PckSize/2
  Mux/1 -> __fcn_ss__/Trigger
  ground/1 -> Mux/2

== system sedemo_ethernet/MAC Controller (B)/Transmission Buffer Controller ==
  #tx : Inport  OutDataType=sfix(16)  OutScaling=2^0
  #success : Inport  Port=2  OutDataType=sfix(16)  OutScaling=2^0
  #failure : Inport  Port=3  OutDataType=sfix(16)  OutScaling=2^0
  Initial Value : simeventssignalmanage1/Initial Value  InitialValue=1
  Transmission Buffer Controller : Subsystem  LoadFcn=des_subsystemblock(gcb, 'load');  InitFcn=des_subsystemblock(gcb, 'init');  StartFcn=des_subsystemblock(gcb, 'start');  StopFcn=des_subsystemblock(gcb, 'stop');
      settings: CopyFcn=des_subsystemblock(gcb, 'copy');  DeleteFcn=des_subsystemblock(gcb, 'delete');  UndoDeleteFcn=des_subsystemblock(gcb, 'undodelete');  ModelCloseFcn=des_subsystemblock(gcb, 'modelclose');  PreSaveFcn=des_subsystemblock(gcb, 'presave');  NameChangeFcn=des_subsystemblock(gcb, 'namechange');  ParentCloseFcn=des_subsystemblock(gcb, 'parentclose');  ErrorFcn=des_error_redirect
  state : Outport  OutDataType=sfix(16)  OutScaling=2^0
  wires:
  Initial Value/1 -> state/1
  Transmission Buffer Controller/1(state) -> Initial Value/1
  #failure/1 -> Transmission Buffer Controller/3(#failure)
  #success/1 -> Transmission Buffer Controller/2(#success)
  #tx/1 -> Transmission Buffer Controller/1(#tx)

== system sedemo_ethernet/MAC Controller (B)/background1 ==

== system sedemo_ethernet/MAC Controller (B)/background2 ==

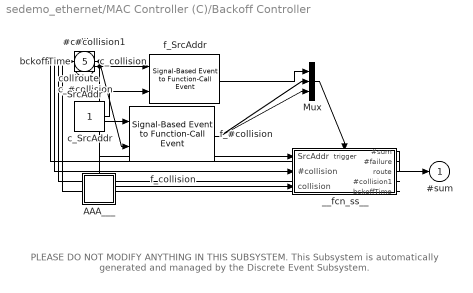
== system sedemo_ethernet/MAC Controller (C)/Backoff Controller ==
  note: PLEASE DO NOT MODIFY ANYTHING IN THIS SUBSYSTEM.
      | This Subsystem is automatically generated and
      | managed by the Discrete Event Subsystem.
  SrcAddr : Inport  DataType=double  OutDataType=sfix(16)  OutScaling=2^0  OutDataTypeStr=double
  #collision : Inport  Port=2  DataType=double  OutDataType=sfix(16)  OutScaling=2^0  OutDataTypeStr=double
  collision : Inport  Port=3  DataType=double  OutDataType=sfix(16)  OutScaling=2^0  OutDataTypeStr=double
  AAA___ : Subsystem  LoadFcn=des_subsystemsupportblock(gcb, 'load');  InitFcn=des_subsystemsupportblock(gcb, 'init');  StartFcn=des_subsystemsupportblock(gcb, 'start');  StopFcn=des_subsystemsupportblock(gcb, 'stop');
      settings: CopyFcn=des_subsystemsupportblock(gcb, 'copy');  DeleteFcn=des_subsystemsupportblock(gcb, 'delete');  UndoDeleteFcn=des_subsystemsupportblock(gcb, 'undodelete');  ModelCloseFcn=des_subsystemsupportblock(gcb, 'modelclose');  PreSaveFcn=des_subsystemsupportblock(gcb, 'presave');  NameChangeFcn=des_subsystemsupportblock(gcb, 'namechange');  OpenFcn=des_subsystemsupportblock(gcb, 'open');  ParentCloseFcn=des_subsystemsupportblock(gcb, 'parentclose');
  Mux : Mux  Inputs=3
  __fcn_ss__ : Subsystem  TreatAsAtomicUnit=on
      settings: PropExecContextOutsideSubsystem=on
  c_#collision : Constant  Value=0  OutDataType=sfix(16)  OutScaling=2^0
  c_SrcAddr : Constant  OutDataType=sfix(16)  OutScaling=2^0
  c_collision : Constant  Value=0  OutDataType=sfix(16)  OutScaling=2^0
  f_#collision : simeventstranslate1/Signal-Based Event to Function-Call Event  Priority=1  SystemSampleTime=-1  GenerateFunctionCallUpon=Sample time hit from port ts  SignalEdgeOption=Rising  EnableE1Port=on  EnableF2Port=off  EnableE2Port=off  SpecifyEventPriority=off  PriorityFunctionCall=20  FunctionCallDelayFrom=Dialog  DelayFunctionCall=0  StatNumberF1Calls=Off  StatNumberF2Calls=Off  MaskBlockType=DESS_DATA_PORT
  f_SrcAddr : simeventstranslate1/Signal-Based Event to Function-Call Event  Priority=1  SystemSampleTime=-1  GenerateFunctionCallUpon=Sample time hit from port ts  SignalEdgeOption=Rising  EnableE1Port=on  EnableF2Port=off  EnableE2Port=off  SpecifyEventPriority=on  PriorityFunctionCall=20  FunctionCallDelayFrom=Dialog  DelayFunctionCall=0  StatNumberF1Calls=Off  StatNumberF2Calls=Off  MaskBlockType=DESS_EVENT_PORT
  f_collision : simeventstranslate1/Signal-Based Event to Function-Call Event  Priority=1  SystemSampleTime=-1  GenerateFunctionCallUpon=Sample time hit from port ts  SignalEdgeOption=Rising  EnableE1Port=on  EnableF2Port=off  EnableE2Port=off  SpecifyEventPriority=off  PriorityFunctionCall=200  FunctionCallDelayFrom=Dialog  DelayFunctionCall=0  StatNumberF1Calls=Off  StatNumberF2Calls=Off  MaskBlockType=DESS_DATA_PORT
  #sum : Outport  OutDataType=sfix(16)  OutScaling=2^0
  #failure : Outport  Port=2  OutDataType=sfix(16)  OutScaling=2^0
  route : Outport  Port=3  OutDataType=sfix(16)  OutScaling=2^0
  #collision1 : Outport  Port=4  OutDataType=sfix(16)  OutScaling=2^0
  bckoffTime : Outport  Port=5  OutDataType=sfix(16)  OutScaling=2^0
  wires:
  SrcAddr/1 -> __fcn_ss__/1(SrcAddr), f_SrcAddr/1
  __fcn_ss__/5(bckoffTime) -> bckoffTime/1
  c_collision/1 -> f_collision/2
  f_collision/1 -> Mux/3
  collision/1 -> __fcn_ss__/3(collision), f_collision/1
  __fcn_ss__/4(#collision1) -> #collision1/1
  __fcn_ss__/3(route) -> route/1
  __fcn_ss__/2(#failure) -> #failure/1
  #collision/1 -> __fcn_ss__/2(#collision), f_#collision/1
  c_#collision/1 -> f_#collision/2
  f_#collision/1 -> Mux/2
  Mux/1 -> __fcn_ss__/Trigger
  c_SrcAddr/1 -> f_SrcAddr/2
  f_SrcAddr/1 -> Mux/1
  __fcn_ss__/1(#sum) -> #sum/1
